simulink model "ASW_OBD"  (R2023a)
settings: configuration reference "cfg_FastTaskCodeGeneration_v01" (kept outside this file)
undefined symbols (not defined in the file): Cdbl_tiSlwTaskSmpTi
(part 1 of 2)
settings Model: DataDictionary=dd_foc_dictionary.sldd  EnableAccessToBaseWorkspace=off  Creator=WFYXQ  LastModifiedBy=xiaoqiang.yuan
settings ConfigSetRef: SourceName=cfg_FastTaskCodeGeneration_v01

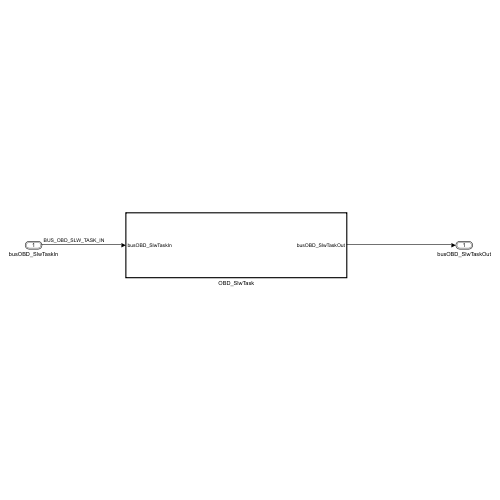
[thumbnail: Simulink's stored preview of the top-level diagram]
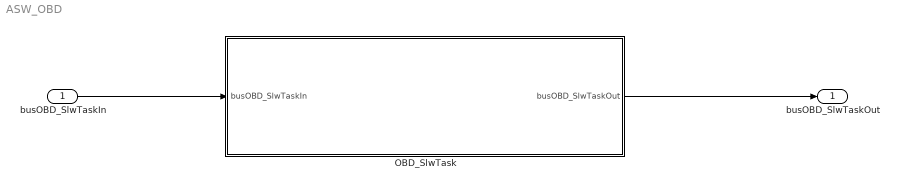
== system ASW_OBD ==
  busOBD_SlwTaskIn : Inport  OutDataTypeStr=Bus: BUS_OBD_SLW_TASK_IN  SampleTime=round(double(Cdbl_tiSlwTaskSmpTi),4)  BusOutputAsStruct=on
  OBD_SlwTask : Subsystem  TreatAsAtomicUnit=on  RTWFcnName=OBD_SlwTask
      settings: RTWSystemCode=Nonreusable function  RTWFcnNameOpts=User specified
  busOBD_SlwTaskOut : Outport  OutDataTypeStr=Bus: BUS_OBD_SLW_TASK_OUT  SampleTime=round(double(Cdbl_tiSlwTaskSmpTi),4)
  wires:
  busOBD_SlwTaskIn/1 -> OBD_SlwTask/1(busOBD_SlwTaskIn)
  OBD_SlwTask/1(busOBD_SlwTaskOut) -> busOBD_SlwTaskOut/1

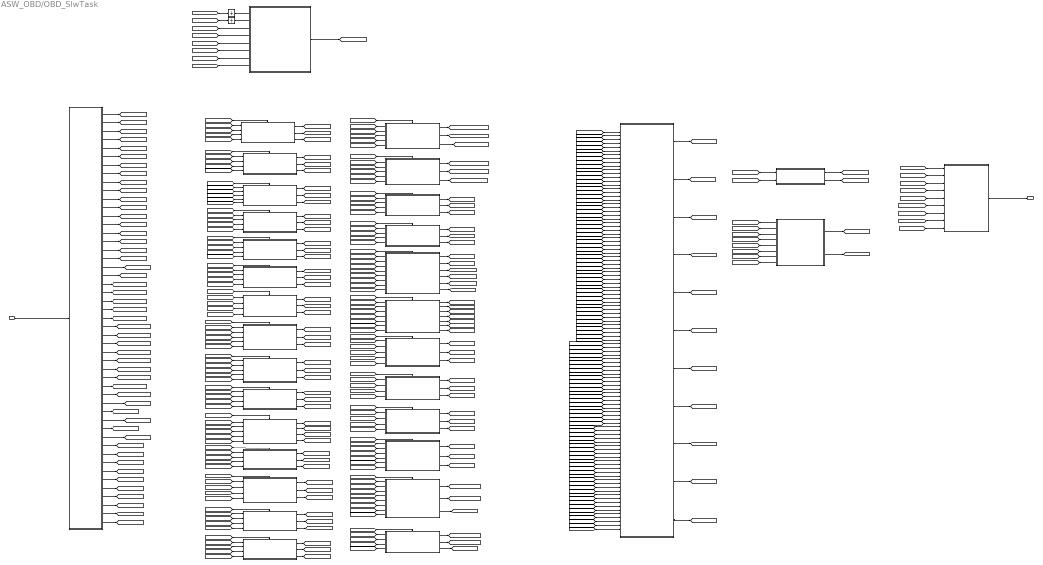
== system ASW_OBD/OBD_SlwTask ==
  note: FaultPreDiagnosis
  busOBD_SlwTaskIn : Inport
  Unit Delay : UnitDelay  SampleTime=-1  HasFrameUpgradeWarning=on
  Unit Delay1 : UnitDelay  SampleTime=-1  HasFrameUpgradeWarning=on
  rss_BattPwrHiLvl1Dia : Subsystem  ReferencedSubsystem=rss_BattPwrHiLvl1Dia
  rss_BusOffFaltDia : Subsystem  ReferencedSubsystem=rss_BusOffFaltDia
  rss_CRASHFaltDia : Subsystem  ReferencedSubsystem=rss_CrashFaltDia
  rss_ChipFaltDia : Subsystem  ReferencedSubsystem=rss_ChipFaltDia
  rss_ComFaltDia : Subsystem  ReferencedSubsystem=rss_ComFaltDia
  rss_CtlBrdVltgHiLvl1Dia : Subsystem  ReferencedSubsystem=rss_CtlBrdVltgHiLvl1Dia
  rss_CtlBrdVltgLoLvl1Dia : Subsystem  ReferencedSubsystem=rss_CtlBrdVltgLoLvl1Dia
  rss_FaltInfoMng : Subsystem  ReferencedSubsystem=rss_FaltInfoMng
  rss_FaltLevlCmpt : Subsystem  ReferencedSubsystem=rss_FaltLevlCmpt
  rss_FaltResp : Subsystem  ReferencedSubsystem=rss_FaltResp
  rss_GDVltgHiLvl1Dia : Subsystem  ReferencedSubsystem=rss_GDVltgHiLvl1Dia
  rss_GDVltgLoLvl1Dia : Subsystem  ReferencedSubsystem=rss_GDVltgLoLvl1Dia
  rss_HWOvrCurrDia : Subsystem  ReferencedSubsystem=rss_HWOvrCurrDia
  rss_MosOpnCirFaltDia : Subsystem  ReferencedSubsystem=rss_MosOpnCirFaltDia
  rss_MotoSpdHiLvl1Dia : Subsystem  ReferencedSubsystem=rss_MotoSpdHiLvl1Dia
  rss_MotoSpdLoLvl1Dia : Subsystem  ReferencedSubsystem=rss_MotoSpdLoLvl1Dia
  rss_MotoTempHiLvl1Dia : Subsystem  ReferencedSubsystem=rss_MotoTempHiLvl1Dia
  rss_MotoTempHiLvl2Dia : Subsystem  ReferencedSubsystem=rss_MotoTempHiLvl2Dia
  rss_MotoTempSensFaltDia : Subsystem  ReferencedSubsystem=rss_MotoTempSensFaltDia
  rss_NoLdDia : Subsystem  ReferencedSubsystem=rss_NoLdDia
  rss_PhCurrHiLvl1Dia : Subsystem  ReferencedSubsystem=rss_PhCurrHiLvl1Dia
  rss_PhCurrSensFaltDia : Subsystem  ReferencedSubsystem=rss_PhCurrSensFaltDia
  rss_PwrTubPCBTempHiLvl1Dia : Subsystem  ReferencedSubsystem=rss_PwrTubPCBTempHiLvl1Dia
  rss_PwrTubPCBTempHiLvl2Dia : Subsystem  ReferencedSubsystem=rss_PwrTubPCBTempHiLvl2Dia
  rss_PwrTubPCBTempSensFaltDia : Subsystem  ReferencedSubsystem=rss_PwrTubPCBTempSensFaltDia
  rss_SplyVltgHiLvl1Dia : Subsystem  ReferencedSubsystem=rss_SplyVltgHiLvl1Dia
  rss_SplyVltgLoLvl1Dia : Subsystem  ReferencedSubsystem=rss_SplyVltgLoLvl1Dia
  rss_SplyVltgLoLvl2Dia : Subsystem  ReferencedSubsystem=rss_SplyVltgLoLvl2Dia
  vrs_FaltEnFlgConf : Subsystem  Variant=on  VariantControlMode=label  VariantControl=Choice  LabelModeActiveChoice=cstSenlCtrlLbl
  vrs_MotoStallDia : Subsystem  Variant=on  VariantControlMode=label  VariantControl=Choice  LabelModeActiveChoice=cstHybrCtrlLbl
  vrs_PhiSensFaltDia : Subsystem  Variant=on  VariantControlMode=label  VariantControl=Choice  LabelModeActiveChoice=cstHybrCtrlLbl
  vrs_SlwTaskIn : Subsystem  Variant=on  VariantControlMode=label  VariantControl=cstSenlCtrlLbl  LabelModeActiveChoice=cstHybrCtrlLbl
  vrs_SlwTaskOut : Subsystem  Variant=on  VariantControlMode=label  VariantControl=Choice  LabelModeActiveChoice=cstHybrCtrlLbl
  busOBD_SlwTaskOut : Outport
  wires:
  vrs_SlwTaskOut/1(busOBD_SlwTaskOut) -> busOBD_SlwTaskOut/1  "busOBD_SlwTaskOut"
  [s16_nRmpRefElecSpd] -> rss_MotoSpdLoLvl1Dia/5
  [s16_nActElecSpd] -> rss_MotoSpdLoLvl1Dia/6
  [enm_stMotoSt] -> rss_MotoSpdLoLvl1Dia/4
  rss_PhCurrHiLvl1Dia/1 -> [bol_flgPhCurrHiLvl1Flg]
  rss_PhCurrHiLvl1Dia/2 -> [bol_flgPhCurrHiLvl1Occ]
  rss_ComFaltDia/1 -> [bol_flgComFaltFlg]
  rss_ComFaltDia/2 -> [bol_flgComFaltOcc]
  rss_BattPwrHiLvl1Dia/1 -> [bol_flgBattPwrHiLvl1Flg]
  rss_NoLdDia/1 -> [bol_flgNoLdFlg]
  rss_SplyVltgHiLvl1Dia/1 -> [bol_flgSplyVltgHiLvl1Flg]
  rss_MotoSpdHiLvl1Dia/1 -> [bol_flgMotoSpdHiLvl1Flg]
  rss_CtlBrdVltgLoLvl1Dia/1 -> [bol_flgCtlBrdVltgLoLvl1Flg]
  rss_FaltInfoMng/1 -> [busOBD_FaltSt]
  [busOBD_FaltSt] -> vrs_SlwTaskOut/1(busOBD_FaltSt)
  [bol_FaltSt] -> rss_FaltLevlCmpt/1
  rss_FaltInfoMng/2 -> [bol_FaltSt]
  [busOBD_FaltSt] -> Unit Delay/1
  [bol_enFaltEnFlg] -> rss_PhCurrHiLvl1Dia/1
  rss_FaltInfoMng/4 -> [u8_stFaltCyclDiaCt]
  rss_FaltInfoMng/5 -> [bol_enFaltRcvEnFlg]
  rss_FaltInfoMng/6 -> [bol_enFaltMngEnFlg]
  [u8_stFaltCyclDiaCt] -> rss_PhCurrHiLvl1Dia/2
  [bol_enFaltRcvEnFlg] -> rss_PhCurrHiLvl1Dia/3
  rss_FaltLevlCmpt/1 -> [u8_stFaltLvl]
  rss_FaltLevlCmpt/2 -> [u8_stMaxFaltLvl]
  rss_FaltInfoMng/7 -> [u8_stFaltLvlCt]
  [u8_stFaltLvlCt] -> rss_FaltLevlCmpt/2
  [u8_stFaltLvl] -> rss_FaltResp/1
  [u8_stMaxFaltLvl] -> rss_FaltResp/2
  rss_FaltResp/1 -> [s16_nFaltRefMechSpd]
  rss_FaltResp/2 -> [s16_trqFaltRefTqLim]
  [u8_ctMotoStallCyclAcc] -> rss_FaltResp/3
  [bol_enFaltEnFlg] -> rss_SplyVltgHiLvl1Dia/1
  [u8_stFaltCyclDiaCt] -> rss_SplyVltgHiLvl1Dia/2
  [bol_enFaltRcvEnFlg] -> rss_SplyVltgHiLvl1Dia/3
  [bol_enFaltEnFlg] -> rss_ComFaltDia/1
  [u8_stFaltCyclDiaCt] -> rss_ComFaltDia/2
  [bol_enFaltRcvEnFlg] -> rss_ComFaltDia/3
  [bol_enFaltEnFlg] -> rss_NoLdDia/1
  [u8_stFaltCyclDiaCt] -> rss_NoLdDia/2
  [bol_enFaltRcvEnFlg] -> rss_NoLdDia/3
  [s16_nActElecSpd] -> rss_NoLdDia/5
  [s16_ampActPhCurrAmp] -> rss_PhCurrHiLvl1Dia/4
  [u16_uSplyVltg] -> rss_SplyVltgHiLvl1Dia/4
  [u8_ctLossNoData] -> rss_ComFaltDia/4
  [u8_ctComRolCnt] -> rss_ComFaltDia/5
  [s16_ampActPhCurrAmp] -> rss_NoLdDia/4
  [bol_enFaltEnFlg] -> rss_MotoSpdLoLvl1Dia/1
  [u8_stFaltCyclDiaCt] -> rss_MotoSpdLoLvl1Dia/2
  [bol_enFaltRcvEnFlg] -> rss_MotoSpdLoLvl1Dia/3
  [u8_ctMotoStallCyclDiaCnt] -> rss_FaltResp/4
  [u8_stMaxFaltLvl] -> vrs_SlwTaskOut/2(u8_stMaxFaltLvl)
  [s16_nFaltRefMechSpd] -> vrs_SlwTaskOut/3(s16_nFaltRefMechSpd)
  [s16_trqFaltRefTqLim] -> vrs_SlwTaskOut/4(s16_trqFaltRefTqLim)
  rss_MotoSpdLoLvl1Dia/1 -> [bol_flgMotoSpdLoLvl1Flg]
  [bol_enFaltEnFlg] -> rss_CtlBrdVltgLoLvl1Dia/1
  [u16_uCtlBrdVltg] -> rss_CtlBrdVltgLoLvl1Dia/4
  [u8_stFaltCyclDiaCt] -> rss_CtlBrdVltgLoLvl1Dia/2
  [bol_enFaltRcvEnFlg] -> rss_CtlBrdVltgLoLvl1Dia/3
  rss_FaltInfoMng/8 -> [bol_flgFstSdlEn]
  rss_FaltInfoMng/9 -> [bol_flgSlwSdlEn]
  [bol_flgFstSdlEn] -> rss_CtlBrdVltgLoLvl1Dia/Enable
  rss_CtlBrdVltgLoLvl1Dia/2 -> [bol_flgCtlBrdVltgLoLvl1Occ]
  [u8_stFaltCyclDiaCt] -> rss_CtlBrdVltgHiLvl1Dia/2
  [bol_flgFstSdlEn] -> rss_CtlBrdVltgHiLvl1Dia/Enable
  [bol_enFaltEnFlg] -> rss_CtlBrdVltgHiLvl1Dia/1
  [bol_enFaltRcvEnFlg] -> rss_CtlBrdVltgHiLvl1Dia/3
  rss_CtlBrdVltgHiLvl1Dia/2 -> [bol_flgCtlBrdVltgHiLvl1Occ]
  rss_CtlBrdVltgHiLvl1Dia/1 -> [bol_flgCtlBrdVltgHiLvl1Flg]
  [u16_uCtlBrdVltg] -> rss_CtlBrdVltgHiLvl1Dia/4
  [bol_flgFstSdlEn] -> rss_PhCurrHiLvl1Dia/Enable
  [bol_flgFstSdlEn] -> rss_HWOvrCurrDia/Enable
  [bol_enFaltEnFlg] -> rss_HWOvrCurrDia/1
  [u8_stFaltCyclDiaCt] -> rss_HWOvrCurrDia/2
  [bol_enFaltRcvEnFlg] -> rss_HWOvrCurrDia/3
  [bol_flgHWOvrCurrFalt] -> rss_HWOvrCurrDia/4
  rss_HWOvrCurrDia/1 -> [bol_flgHWOvrCurrFlg]
  rss_HWOvrCurrDia/2 -> [bol_flgHWOvrCurrOcc]
  [bol_flgFstSdlEn] -> rss_SplyVltgLoLvl1Dia/Enable
  [bol_enFaltEnFlg] -> rss_SplyVltgLoLvl1Dia/1
  [u8_stFaltCyclDiaCt] -> rss_SplyVltgLoLvl1Dia/2
  [bol_enFaltRcvEnFlg] -> rss_SplyVltgLoLvl1Dia/3
  [u16_uSplyVltg] -> rss_SplyVltgLoLvl1Dia/4
  rss_SplyVltgLoLvl1Dia/1 -> [bol_flgSplyVltgLoLvl1Flg]
  rss_SplyVltgLoLvl1Dia/2 -> [bol_flgSplyVltgLoLvl1Occ]
  [bol_flgFstSdlEn] -> rss_SplyVltgLoLvl2Dia/Enable
  [bol_enFaltEnFlg] -> rss_SplyVltgLoLvl2Dia/1
  [u8_stFaltCyclDiaCt] -> rss_SplyVltgLoLvl2Dia/2
  [bol_enFaltRcvEnFlg] -> rss_SplyVltgLoLvl2Dia/3
  [u16_uSplyVltg] -> rss_SplyVltgLoLvl2Dia/4
  rss_SplyVltgLoLvl2Dia/1 -> [bol_flgSplyVltgLoLvl2Flg]
  rss_SplyVltgLoLvl2Dia/2 -> [bol_flgSplyVltgLoLvl2Occ]
  [bol_flgFstSdlEn] -> rss_SplyVltgHiLvl1Dia/Enable
  rss_SplyVltgHiLvl1Dia/2 -> [bol_flgSplyVltgHiLvl1Occ]
  [bol_enFaltEnFlg] -> rss_PwrTubPCBTempHiLvl1Dia/1
  [u8_stFaltCyclDiaCt] -> rss_PwrTubPCBTempHiLvl1Dia/2
  [bol_enFaltRcvEnFlg] -> rss_PwrTubPCBTempHiLvl1Dia/3
  [u8_tPwrTubTemp] -> rss_PwrTubPCBTempHiLvl1Dia/4
  [u8_tPCBTempSubs] -> rss_PwrTubPCBTempHiLvl1Dia/5
  [bol_flgSlwSdlEn] -> rss_PwrTubPCBTempHiLvl1Dia/Enable
  rss_PwrTubPCBTempHiLvl1Dia/1 -> [bol_flgPwrTubPCBTempHiLvl1Flg]
  rss_PwrTubPCBTempHiLvl1Dia/2 -> [bol_flgPwrTubPCBTempHiLvl1Occ]
  [bol_flgSlwSdlEn] -> rss_PwrTubPCBTempHiLvl2Dia/Enable
  [bol_enFaltEnFlg] -> rss_PwrTubPCBTempHiLvl2Dia/1
  [u8_stFaltCyclDiaCt] -> rss_PwrTubPCBTempHiLvl2Dia/2
  [bol_enFaltRcvEnFlg] -> rss_PwrTubPCBTempHiLvl2Dia/3
  [u8_tPwrTubTemp] -> rss_PwrTubPCBTempHiLvl2Dia/4
  [u8_tPCBTempSubs] -> rss_PwrTubPCBTempHiLvl2Dia/5
  rss_PwrTubPCBTempHiLvl2Dia/1 -> [bol_flgPwrTubPCBTempHiLvl2Flg]
  rss_PwrTubPCBTempHiLvl2Dia/2 -> [bol_flgPwrTubPCBTempHiLvl2Occ]
  [bol_enFaltEnFlg] -> rss_MotoTempHiLvl1Dia/1
  [u8_stFaltCyclDiaCt] -> rss_MotoTempHiLvl1Dia/2
  [bol_enFaltRcvEnFlg] -> rss_MotoTempHiLvl1Dia/3
  [u8_tMotoTemp] -> rss_MotoTempHiLvl1Dia/4
  [bol_flgSlwSdlEn] -> rss_MotoTempHiLvl1Dia/Enable
  rss_MotoTempHiLvl1Dia/1 -> [bol_flgMotoTempHiLvl1Flg]
  rss_MotoTempHiLvl1Dia/2 -> [bol_flgMotoTempHiLvl1Occ]
  [u8_tMotoTemp] -> rss_MotoTempHiLvl2Dia/4
  [bol_flgSlwSdlEn] -> rss_MotoTempHiLvl2Dia/Enable
  [u8_stFaltCyclDiaCt] -> rss_MotoTempHiLvl2Dia/2
  rss_MotoTempHiLvl2Dia/1 -> [bol_flgMotoTempHiLvl2Flg]
  [bol_enFaltEnFlg] -> rss_MotoTempHiLvl2Dia/1
  [bol_enFaltRcvEnFlg] -> rss_MotoTempHiLvl2Dia/3
  rss_MotoTempHiLvl2Dia/2 -> [bol_flgMotoTempHiLvl2Occ]
  [bol_flgFstSdlEn] -> rss_NoLdDia/Enable
  rss_NoLdDia/2 -> [bol_flgNoLdOcc]
  [s16_pwrSplyElecPwr] -> rss_BattPwrHiLvl1Dia/4
  [bol_enFaltEnFlg] -> rss_BattPwrHiLvl1Dia/1
  [u8_stFaltCyclDiaCt] -> rss_BattPwrHiLvl1Dia/2
  [bol_enFaltRcvEnFlg] -> rss_BattPwrHiLvl1Dia/3
  [bol_flgSlwSdlEn] -> rss_BattPwrHiLvl1Dia/Enable
  rss_BattPwrHiLvl1Dia/2 -> [bol_flgBattPwrHiLvl1Occ]
  rss_MotoSpdLoLvl1Dia/2 -> [bol_flgMotoSpdLoLvl1Occ]
  [bol_flgSlwSdlEn] -> rss_MotoSpdLoLvl1Dia/Enable
  rss_MotoSpdHiLvl1Dia/2 -> [bol_flgMotoSpdHiLvl1Occ]
  [bol_enFaltRcvEnFlg] -> rss_MotoSpdHiLvl1Dia/3
  [u8_stFaltCyclDiaCt] -> rss_MotoSpdHiLvl1Dia/2
  [bol_enFaltEnFlg] -> rss_MotoSpdHiLvl1Dia/1
  [bol_flgSlwSdlEn] -> rss_MotoSpdHiLvl1Dia/Enable
  [s16_nActElecSpd] -> rss_MotoSpdHiLvl1Dia/4
  [bol_flgGDVltgHiLvl1] -> rss_GDVltgHiLvl1Dia/4
  rss_GDVltgHiLvl1Dia/1 -> [bol_flgGDVltgHiLvl1Flg]
  rss_GDVltgHiLvl1Dia/2 -> [bol_flgGDVltgHiLvl1Occ]
  [bol_enFaltRcvEnFlg] -> rss_GDVltgHiLvl1Dia/3
  [bol_enFaltEnFlg] -> rss_GDVltgHiLvl1Dia/1
  [bol_flgFstSdlEn] -> rss_GDVltgHiLvl1Dia/Enable
  [u8_stFaltCyclDiaCt] -> rss_GDVltgHiLvl1Dia/2
  rss_GDVltgLoLvl1Dia/2 -> [bol_flgGDVltgLoLvl1Occ]
  [bol_flgFstSdlEn] -> rss_GDVltgLoLvl1Dia/Enable
  [bol_enFaltRcvEnFlg] -> rss_GDVltgLoLvl1Dia/3
  [u8_stFaltCyclDiaCt] -> rss_GDVltgLoLvl1Dia/2
  [bol_flgGDVltgLoLvl1] -> rss_GDVltgLoLvl1Dia/4
  [bol_enFaltEnFlg] -> rss_GDVltgLoLvl1Dia/1
  rss_GDVltgLoLvl1Dia/1 -> [bol_flgGDVltgLoLvl1Flg]
  rss_ChipFaltDia/1 -> [bol_flgChipFaltFlg]
  [bol_enFaltEnFlg] -> rss_ChipFaltDia/1
  [u8_stFaltCyclDiaCt] -> rss_ChipFaltDia/2
  [bol_enFaltRcvEnFlg] -> rss_ChipFaltDia/3
  [bol_flgChipFalt] -> rss_ChipFaltDia/4
  [bol_flgFstSdlEn] -> rss_ChipFaltDia/Enable
  rss_ChipFaltDia/2 -> [bol_flgChipFaltOcc]
  [u16_uADActPhCurr] -> rss_PhCurrSensFaltDia/4
  [bol_flgFstSdlEn] -> rss_PhCurrSensFaltDia/Enable
  [bol_enFaltEnFlg] -> rss_PhCurrSensFaltDia/1
  [u8_stFaltCyclDiaCt] -> rss_PhCurrSensFaltDia/2
  [bol_enFaltRcvEnFlg] -> rss_PhCurrSensFaltDia/3
  rss_PhCurrSensFaltDia/1 -> [bol_flgPhCurrSensFaltFlg]
  rss_PhCurrSensFaltDia/2 -> [bol_flgPhCurrSensFaltOcc]
  rss_PwrTubPCBTempSensFaltDia/1 -> [bol_flgPwrTubPCBTempSensFaltFlg]
  rss_PwrTubPCBTempSensFaltDia/2 -> [bol_flgPwrTubPCBTempSensFaltOcc]
  [bol_flgSlwSdlEn] -> rss_PwrTubPCBTempSensFaltDia/Enable
  [bol_enFaltEnFlg] -> rss_PwrTubPCBTempSensFaltDia/1
  [u8_stFaltCyclDiaCt] -> rss_PwrTubPCBTempSensFaltDia/2
  [bol_enFaltRcvEnFlg] -> rss_PwrTubPCBTempSensFaltDia/3
  [u16_uADPwrTubTemp] -> rss_PwrTubPCBTempSensFaltDia/4
  [u16_uADPCBTemp] -> rss_PwrTubPCBTempSensFaltDia/5
  [u16_uADMotoTemp] -> rss_MotoTempSensFaltDia/4
  [bol_enFaltRcvEnFlg] -> rss_MotoTempSensFaltDia/3
  [u8_stFaltCyclDiaCt] -> rss_MotoTempSensFaltDia/2
  [bol_enFaltEnFlg] -> rss_MotoTempSensFaltDia/1
  [bol_flgSlwSdlEn] -> rss_MotoTempSensFaltDia/Enable
  rss_MotoTempSensFaltDia/1 -> [bol_flgMotoTempSensFaltFlg]
  rss_MotoTempSensFaltDia/2 -> [bol_flgMotoTempSensFaltOcc]
  [bol_flgComSdlEn] -> rss_ComFaltDia/Enable
  [bol_flgPhCurrHiLvl1Flg] -> rss_FaltInfoMng/1
  [bol_flgHWOvrCurrFlg] -> rss_FaltInfoMng/2
  [bol_flgSplyVltgLoLvl1Flg] -> rss_FaltInfoMng/3
  [bol_flgSplyVltgLoLvl2Flg] -> rss_FaltInfoMng/4
  [bol_flgSplyVltgHiLvl1Flg] -> rss_FaltInfoMng/5
  [bol_flgPwrTubPCBTempHiLvl1Flg] -> rss_FaltInfoMng/6
  [bol_flgPwrTubPCBTempHiLvl2Flg] -> rss_FaltInfoMng/7
  [bol_flgMotoTempHiLvl1Flg] -> rss_FaltInfoMng/8
  [bol_flgMotoTempHiLvl2Flg] -> rss_FaltInfoMng/9
  [bol_flgComFaltFlg] -> rss_FaltInfoMng/10
  [bol_flgMotoStallPermFlg] -> rss_FaltInfoMng/11
  [bol_flgMotoStallTmpFlg] -> rss_FaltInfoMng/12
  [bol_flgNoLdFlg] -> rss_FaltInfoMng/13
  [bol_flgBattPwrHiLvl1Flg] -> rss_FaltInfoMng/14
  [bol_flgMotoSpdHiLvl1Flg] -> rss_FaltInfoMng/15
  [bol_flgMotoSpdLoLvl1Flg] -> rss_FaltInfoMng/16
  [bol_flgCtlBrdVltgLoLvl1Flg] -> rss_FaltInfoMng/17
  [bol_flgCtlBrdVltgHiLvl1Flg] -> rss_FaltInfoMng/18
  [bol_flgGDVltgLoLvl1Flg] -> rss_FaltInfoMng/19
  [bol_flgGDVltgHiLvl1Flg] -> rss_FaltInfoMng/20
  [bol_flgChipFaltFlg] -> rss_FaltInfoMng/21
  [bol_flgPhiSensFaltFlg] -> rss_FaltInfoMng/22
  [bol_flgPhCurrSensFaltFlg] -> rss_FaltInfoMng/23
  [bol_flgPwrTubPCBTempSensFaltFlg] -> rss_FaltInfoMng/24
  [bol_flgMotoTempSensFaltFlg] -> rss_FaltInfoMng/25
  [bol_flgPhCurrHiLvl1Occ] -> rss_FaltInfoMng/29
  [bol_flgHWOvrCurrOcc] -> rss_FaltInfoMng/30
  [bol_flgSplyVltgLoLvl1Occ] -> rss_FaltInfoMng/31
  [bol_flgSplyVltgLoLvl2Occ] -> rss_FaltInfoMng/32
  [bol_flgSplyVltgHiLvl1Occ] -> rss_FaltInfoMng/33
  [bol_flgPwrTubPCBTempHiLvl1Occ] -> rss_FaltInfoMng/34
  [bol_flgPwrTubPCBTempHiLvl2Occ] -> rss_FaltInfoMng/35
  [bol_flgMotoTempHiLvl1Occ] -> rss_FaltInfoMng/36
  [bol_flgMotoTempHiLvl2Occ] -> rss_FaltInfoMng/37
  [bol_flgComFaltOcc] -> rss_FaltInfoMng/38
  [bol_flgMotoStallOcc] -> rss_FaltInfoMng/39
  [bol_flgMotoStallOcc] -> rss_FaltInfoMng/40
  [bol_flgNoLdOcc] -> rss_FaltInfoMng/41
  [bol_flgBattPwrHiLvl1Occ] -> rss_FaltInfoMng/42
  [bol_flgMotoSpdHiLvl1Occ] -> rss_FaltInfoMng/43
  [bol_flgMotoSpdLoLvl1Occ] -> rss_FaltInfoMng/44
  [bol_flgCtlBrdVltgLoLvl1Occ] -> rss_FaltInfoMng/45
  [bol_flgCtlBrdVltgHiLvl1Occ] -> rss_FaltInfoMng/46
  [bol_flgGDVltgLoLvl1Occ] -> rss_FaltInfoMng/47
  [bol_flgGDVltgHiLvl1Occ] -> rss_FaltInfoMng/48
  [bol_flgChipFaltOcc] -> rss_FaltInfoMng/49
  [bol_flgPhiSensFaltOcc] -> rss_FaltInfoMng/50
  [bol_flgPhCurrSensFaltOcc] -> rss_FaltInfoMng/51
  [bol_flgPwrTubPCBTempSensFaltOcc] -> rss_FaltInfoMng/52
  [bol_flgMotoTempSensFaltOcc] -> rss_FaltInfoMng/53
  rss_FaltInfoMng/3 -> [bus_FaltStOcc]
  [bus_FaltStOcc] -> Unit Delay1/1
  [busOBD_FaltSt] -> rss_FaltResp/5
  [bol_flgSlwSdlEn] -> rss_FaltResp/6
  [u16_uSplyVltg] -> rss_FaltInfoMng/57
  [s16_nRmpRefElecSpd] -> rss_FaltInfoMng/58
  [u8_tPCBTemp] -> rss_FaltInfoMng/59
  [u8_tMotoTemp] -> rss_FaltInfoMng/60
  [u8_tPwrTubTemp] -> rss_FaltInfoMng/61
  [u16_uCtlBrdVltg] -> rss_FaltInfoMng/62
  [s16_iActPhCurr] -> rss_FaltInfoMng/63
  [enm_stMotoSt] -> rss_FaltInfoMng/64
  [s16_iEstSplyCurr] -> rss_FaltInfoMng/65
  [s16_iRefDaxQaxCurr] -> rss_FaltInfoMng/66
  [s16_iActDaxQaxCurr] -> rss_FaltInfoMng/67
  [s16_nActElecSpd] -> rss_FaltInfoMng/68
  [bol_flgShOffFlg] -> rss_FaltInfoMng/69
  [bol_enFaltInfoClrUDS14] -> rss_FaltInfoMng/70
  [u16_vVehSpd] -> rss_FaltInfoMng/71
  [u32_disOde] -> rss_FaltInfoMng/72
  [u32_tiStamHi] -> rss_FaltInfoMng/73
  [u32_tiStamLo] -> rss_FaltInfoMng/74
  [u8_psiOilFlow] -> rss_FaltInfoMng/75
  [u8_tOilTemp] -> rss_FaltInfoMng/76
  [bol_enPosSCDCalibEnFlg] -> rss_FaltInfoMng/77
  [u8_psiUpLimOilFlow] -> rss_FaltInfoMng/78
  [bol_flgFstSdlEn] -> rss_BusOffFaltDia/Enable
  [bol_flgBusOffFaltRaw] -> rss_BusOffFaltDia/4
  [bol_enFaltRcvEnFlg] -> rss_BusOffFaltDia/3
  [u8_stFaltCyclDiaCt] -> rss_BusOffFaltDia/2
  [bol_enFaltEnFlg] -> rss_BusOffFaltDia/1
  rss_BusOffFaltDia/2 -> [bol_flgBusOffFaltOcc]
  rss_BusOffFaltDia/1 -> [bol_flgBusOffFaltFlg]
  [bol_flgBusOffFaltOcc] -> rss_FaltInfoMng/54
  [bol_flgBusOffFaltFlg] -> rss_FaltInfoMng/26
  [bol_flgCRCFaltRaw] -> rss_ComFaltDia/6
  [bol_flgMesgLngthFaltRaw] -> rss_ComFaltDia/7
  [s16_nComRefMechSpd] -> rss_ComFaltDia/8
  rss_FaltInfoMng/10 -> [bol_flgComSdlEn]
  [bol_enFaltEnFlg] -> vrs_MotoStallDia/1(bol_enFaltEnFlg)
  [u8_stFaltCyclDiaCt] -> vrs_MotoStallDia/2(u8_stFaltCyclDiaCt)
  [bol_enFaltRcvEnFlg] -> vrs_MotoStallDia/3(bol_enFaltRcvEnFlg)
  [s16_nRmpRefElecSpd] -> vrs_MotoStallDia/4(s16_nRmpRefElecSpd)
  [s16_nActElecSpd] -> vrs_MotoStallDia/5(s16_nActElecSpd)
  [bol_flgFstSdlEn] -> vrs_MotoStallDia/Enable
  vrs_MotoStallDia/1(bol_flgMotoStallTmpFlg) -> [bol_flgMotoStallTmpFlg]
  vrs_MotoStallDia/2(bol_flgMotoStallPermFlg) -> [bol_flgMotoStallPermFlg]
  vrs_MotoStallDia/3(u8_ctMotoStallCyclAcc) -> [u8_ctMotoStallCyclAcc]
  vrs_MotoStallDia/4(bol_flgMotoStallOcc) -> [bol_flgMotoStallOcc]
  vrs_MotoStallDia/5(u8_ctMotoStallCyclDiaCnt) -> [u8_ctMotoStallCyclDiaCnt]
  [u16_psiEstPermMagFlx] -> vrs_MotoStallDia/6(u16_psiEstPermMagFlx)
  Unit Delay/1 -> vrs_FaltEnFlgConf/1(busOBD_FaltSt)
  Unit Delay1/1 -> vrs_FaltEnFlgConf/2(bus_FaltStOcc)
  [bol_enFaltMngEnFlg] -> vrs_FaltEnFlgConf/3(bol_enFaltMngEnFlg)
  [enm_stSysSt] -> vrs_FaltEnFlgConf/4(enm_stSysSt)
  [s16_nComRefMechSpd] -> vrs_FaltEnFlgConf/5(s16_nComRefMechSpd)
  [bol_flgFaltEnFlgUDS85] -> vrs_FaltEnFlgConf/6(bol_flgFaltEnFlgUDS85)
  [bol_flgWBSSt] -> vrs_FaltEnFlgConf/7(bol_flgWBSSt)
  [u16_uCtlBrdVltg] -> vrs_FaltEnFlgConf/8(u16_uCtlBrdVltg)
  vrs_FaltEnFlgConf/1(bol_enFaltEnFlg) -> [bol_enFaltEnFlg]
  busOBD_SlwTaskIn/1 -> vrs_SlwTaskIn/1(busOBD_SlwTaskIn)  "busOBD_SlwTaskIn"
  vrs_SlwTaskIn/1(s16_nRmpRefElecSpd) -> [s16_nRmpRefElecSpd]
  vrs_SlwTaskIn/2(s16_nActElecSpd) -> [s16_nActElecSpd]
  vrs_SlwTaskIn/3(enm_stMotoSt) -> [enm_stMotoSt]
  vrs_SlwTaskIn/4(s16_ampActPhCurrAmp) -> [s16_ampActPhCurrAmp]
  vrs_SlwTaskIn/5(u16_uSplyVltg) -> [u16_uSplyVltg]
  vrs_SlwTaskIn/6(u8_tPwrTubTemp) -> [u8_tPwrTubTemp]
  vrs_SlwTaskIn/7(u8_tPCBTemp) -> [u8_tPCBTemp]
  vrs_SlwTaskIn/8(u8_tMotoTemp) -> [u8_tMotoTemp]
  vrs_SlwTaskIn/9(u8_ctLossNoData) -> [u8_ctLossNoData]
  vrs_SlwTaskIn/10(u8_ctComRolCnt) -> [u8_ctComRolCnt]
  vrs_SlwTaskIn/11(u16_uCtlBrdVltg) -> [u16_uCtlBrdVltg]
  vrs_SlwTaskIn/12(enm_stSysSt) -> [enm_stSysSt]
  vrs_SlwTaskIn/13(bol_flgHWOvrCurrFalt) -> [bol_flgHWOvrCurrFalt]
  vrs_SlwTaskIn/14(bol_flgChipFalt) -> [bol_flgChipFalt]
  vrs_SlwTaskIn/15(bol_flgPhiSensFalt) -> [bol_flgPhiSensFalt]
  vrs_SlwTaskIn/16(u16_uADActPhCurr) -> [u16_uADActPhCurr]
  vrs_SlwTaskIn/17(u16_uADPwrTubTemp) -> [u16_uADPwrTubTemp]
  vrs_SlwTaskIn/18(u16_uADPCBTemp) -> [u16_uADPCBTemp]
  vrs_SlwTaskIn/19(u16_uADMotoTemp) -> [u16_uADMotoTemp]
  vrs_SlwTaskIn/20(s16_pwrSplyElecPwr) -> [s16_pwrSplyElecPwr]
  vrs_SlwTaskIn/21(s16_iActPhCurr) -> [s16_iActPhCurr]
  vrs_SlwTaskIn/22(s16_iEstSplyCurr) -> [s16_iEstSplyCurr]
  vrs_SlwTaskIn/23(s16_iRefDaxQaxCurr) -> [s16_iRefDaxQaxCurr]
  vrs_SlwTaskIn/24(s16_iActDaxQaxCurr) -> [s16_iActDaxQaxCurr]
  vrs_SlwTaskIn/25(bol_flgShOffFlg) -> [bol_flgShOffFlg]
  vrs_SlwTaskIn/26(bol_enFaltInfoClrUDS14) -> [bol_enFaltInfoClrUDS14]
  vrs_SlwTaskIn/27(u16_vVehSpd) -> [u16_vVehSpd]
  vrs_SlwTaskIn/28(u32_disOde) -> [u32_disOde]
  vrs_SlwTaskIn/29(u32_tiStamHi) -> [u32_tiStamHi]
  vrs_SlwTaskIn/30(u32_tiStamLo) -> [u32_tiStamLo]
  vrs_SlwTaskIn/31(u8_psiOilFlow) -> [u8_psiOilFlow]
  vrs_SlwTaskIn/32(u8_tOilTemp) -> [u8_tOilTemp]
  vrs_SlwTaskIn/33(bol_enPosSCDCalibEnFlg) -> [bol_enPosSCDCalibEnFlg]
  vrs_SlwTaskIn/34(u8_psiUpLimOilFlow) -> [u8_psiUpLimOilFlow]
  vrs_SlwTaskIn/35(bol_flgBusOffFaltRaw) -> [bol_flgBusOffFaltRaw]
  vrs_SlwTaskIn/36(bol_flgFaltEnFlgUDS85) -> [bol_flgFaltEnFlgUDS85]
  vrs_SlwTaskIn/37(bol_flgWBSSt) -> [bol_flgWBSSt]
  vrs_SlwTaskIn/38(bol_flgCRCFaltRaw) -> [bol_flgCRCFaltRaw]
  vrs_SlwTaskIn/39(bol_flgMesgLngthFaltRaw) -> [bol_flgMesgLngthFaltRaw]
  vrs_SlwTaskIn/40(s16_nComRefMechSpd) -> [s16_nComRefMechSpd]
  vrs_SlwTaskIn/41(u16_psiEstPermMagFlx) -> [u16_psiEstPermMagFlx]
  [bol_enFaltEnFlg] -> vrs_PhiSensFaltDia/1(bol_enFaltEnFlg)
  [u8_stFaltCyclDiaCt] -> vrs_PhiSensFaltDia/2(u8_stFaltCyclDiaCt)
  [bol_enFaltRcvEnFlg] -> vrs_PhiSensFaltDia/3(bol_enFaltRcvEnFlg)
  [bol_flgPhiSensFalt] -> vrs_PhiSensFaltDia/4(bol_flgPhiSensFalt)
  [bol_flgFstSdlEn] -> vrs_PhiSensFaltDia/Enable
  vrs_PhiSensFaltDia/1(bol_flgPhiSensFaltFlg) -> [bol_flgPhiSensFaltFlg]
  vrs_PhiSensFaltDia/2(bol_flgPhiSensFaltOcc) -> [bol_flgPhiSensFaltOcc]
  vrs_PhiSensFaltDia/3(bol_flgPhiSensFaltRawFlg) -> [bol_flgPhiSensFaltRawFlg]
  [enm_modeAgEvalMode] -> vrs_PhiSensFaltDia/5(enm_modeAgEvalMode)
  [enm_modeAgEvalMode] -> vrs_MotoStallDia/7(enm_modeAgEvalMode)
  [bol_flgPhiSensFaltRawFlg] -> vrs_SlwTaskOut/5(bol_flgPhiSensFaltRawFlg)
  vrs_SlwTaskIn/42(enm_modeAgEvalMode) -> [enm_modeAgEvalMode]
  [enm_stSysSt] -> rss_FaltResp/7
  [bol_enFaltRcvEnFlg] -> rss_CRASHFaltDia/3
  [bol_flgCrashFalt] -> rss_CRASHFaltDia/4
  [u8_stFaltCyclDiaCt] -> rss_CRASHFaltDia/2
  [bol_enFaltEnFlg] -> rss_CRASHFaltDia/1
  [bol_flgFstSdlEn] -> rss_CRASHFaltDia/Enable
  rss_CRASHFaltDia/1 -> [bol_flgCrashFaltFlg]
  rss_CRASHFaltDia/2 -> [bol_flgCrashFaltOcc]
  [bol_flgCrashFaltFlg] -> rss_FaltInfoMng/27
  [bol_flgCrashFaltOcc] -> rss_FaltInfoMng/55
  [u16_uSplyVltg] -> rss_FaltResp/8
  vrs_SlwTaskIn/43(bol_flgCrashFalt) -> [bol_flgCrashFalt]
  vrs_SlwTaskIn/45(bol_flgGDVltgLoLvl1) -> [bol_flgGDVltgLoLvl1]
  vrs_SlwTaskIn/44(bol_flgGDVltgHiLvl1) -> [bol_flgGDVltgHiLvl1]
  [u8_tPwrTubTemp] -> rss_PwrTubPCBTempSensFaltDia/6
  [u8_tPCBTemp] -> rss_PwrTubPCBTempSensFaltDia/7
  [u8_tMCUTemp] -> rss_PwrTubPCBTempSensFaltDia/8
  vrs_SlwTaskIn/46(u8_tMCUTemp) -> [u8_tMCUTemp]
  vrs_SlwTaskIn/47(u8_tPCBTempSubs) -> [u8_tPCBTempSubs]
  [u16_uGDVltg] -> rss_GDVltgHiLvl1Dia/5
  [u16_uGDVltg] -> rss_GDVltgLoLvl1Dia/5
  vrs_SlwTaskIn/48(u16_uGDVltg) -> [u16_uGDVltg]
  rss_ComFaltDia/3 -> [bol_flgComNodeLosFaltDeb]
  rss_ComFaltDia/4 -> [bol_flgComRolCntFaltDeb]
  rss_ComFaltDia/5 -> [bol_flgCRCFaltDeb]
  [bol_flgComNodeLosFaltDeb] -> vrs_SlwTaskOut/6(bol_flgComNodeLosFaltDeb)
  [bol_flgComRolCntFaltDeb] -> vrs_SlwTaskOut/7(bol_flgComRolCntFaltDeb)
  [bol_flgCRCFaltDeb] -> vrs_SlwTaskOut/8(bol_flgCRCFaltDeb)
  [bol_flgMosOpnCirFalt] -> rss_MosOpnCirFaltDia/4
  [bol_enFaltEnFlg] -> rss_MosOpnCirFaltDia/1
  [bol_enFaltRcvEnFlg] -> rss_MosOpnCirFaltDia/3
  rss_MosOpnCirFaltDia/1 -> [bol_flgMosOpnCirFaltFlg]
  rss_MosOpnCirFaltDia/2 -> [bol_flgMosOpnCirFaltOcc]
  [u8_stFaltCyclDiaCt] -> rss_MosOpnCirFaltDia/2
  [bol_flgFstSdlEn] -> rss_MosOpnCirFaltDia/Enable
  [bol_flgMosOpnCirFaltFlg] -> rss_FaltInfoMng/28
  [bol_flgMosOpnCirFaltOcc] -> rss_FaltInfoMng/56
  [bol_flgPhCurrHiLvl1Tmp] -> rss_FaltInfoMng/79
  [bol_flgHWOvrCurrTmp] -> rss_FaltInfoMng/80
  [bol_flgSplyVltgLoLvl1Tmp] -> rss_FaltInfoMng/81
  [bol_flgSplyVltgLoLvl2Tmp] -> rss_FaltInfoMng/82
  [bol_flgSplyVltgHiLvl1Tmp] -> rss_FaltInfoMng/83
  [bol_flgPwrTubPCBTempHiLvl1Tmp] -> rss_FaltInfoMng/84
  [bol_flgPwrTubPCBTempHiLvl2Tmp] -> rss_FaltInfoMng/85
  [bol_flgMotoTempHiLvl1Tmp] -> rss_FaltInfoMng/86
  [bol_flgMotoTempHiLvl2Tmp] -> rss_FaltInfoMng/87
  [bol_flgComFaltTmp] -> rss_FaltInfoMng/88
  [bol_flgMotoStallPermTmp] -> rss_FaltInfoMng/89
  [bol_flgMotoStallTmpTmp] -> rss_FaltInfoMng/90
  [bol_flgNoLdTmp] -> rss_FaltInfoMng/91
  [bol_flgBattPwrHiLvl1Tmp] -> rss_FaltInfoMng/92
  [bol_flgMotoSpdHiLvl1Tmp] -> rss_FaltInfoMng/93
  [bol_flgMotoSpdLoLvl1Tmp] -> rss_FaltInfoMng/94
  [bol_flgCtlBrdVltgLoLvl1Tmp] -> rss_FaltInfoMng/95
  [bol_flgCtlBrdVltgHiLvl1Tmp] -> rss_FaltInfoMng/96
  [bol_flgGDVltgLoLvl1Tmp] -> rss_FaltInfoMng/97
  [bol_flgGDVltgHiLvl1Tmp] -> rss_FaltInfoMng/98
  [bol_flgChipFaltTmp] -> rss_FaltInfoMng/99
  [bol_flgPhiSensFaltTmp] -> rss_FaltInfoMng/100
  [bol_flgPhCurrSensFaltTmp] -> rss_FaltInfoMng/101
  [bol_flgPwrTubPCBTempSensFaltTmp] -> rss_FaltInfoMng/102
  [bol_flgMotoTempSensFaltTmp] -> rss_FaltInfoMng/103
  [bol_flgBusOffFaltTmp] -> rss_FaltInfoMng/104
  [bol_flgCrashFaltTmp] -> rss_FaltInfoMng/105
  [bol_flgMosOpnCirFaltTmp] -> rss_FaltInfoMng/106
  rss_CtlBrdVltgLoLvl1Dia/3 -> [bol_flgCtlBrdVltgLoLvl1Tmp]
  rss_PhCurrHiLvl1Dia/3 -> [bol_flgPhCurrHiLvl1Tmp]
  rss_HWOvrCurrDia/3 -> [bol_flgHWOvrCurrTmp]
  rss_SplyVltgLoLvl1Dia/3 -> [bol_flgSplyVltgLoLvl1Tmp]
  rss_SplyVltgLoLvl2Dia/3 -> [bol_flgSplyVltgLoLvl2Tmp]
  rss_SplyVltgHiLvl1Dia/3 -> [bol_flgSplyVltgHiLvl1Tmp]
  rss_CtlBrdVltgHiLvl1Dia/3 -> [bol_flgCtlBrdVltgHiLvl1Tmp]
  rss_GDVltgLoLvl1Dia/3 -> [bol_flgGDVltgLoLvl1Tmp]
  rss_GDVltgHiLvl1Dia/3 -> [bol_flgGDVltgHiLvl1Tmp]
  rss_ChipFaltDia/3 -> [bol_flgChipFaltTmp]
  vrs_PhiSensFaltDia/4(bol_flgPhiSensFaltTmp) -> [bol_flgPhiSensFaltTmp]
  rss_PhCurrSensFaltDia/3 -> [bol_flgPhCurrSensFaltTmp]
  rss_BusOffFaltDia/3 -> [bol_flgBusOffFaltTmp]
  rss_CRASHFaltDia/3 -> [bol_flgCrashFaltTmp]
  rss_MosOpnCirFaltDia/3 -> [bol_flgMosOpnCirFaltTmp]
  rss_PwrTubPCBTempHiLvl1Dia/3 -> [bol_flgPwrTubPCBTempHiLvl1Tmp]
  rss_PwrTubPCBTempHiLvl2Dia/3 -> [bol_flgPwrTubPCBTempHiLvl2Tmp]
  rss_MotoTempHiLvl1Dia/3 -> [bol_flgMotoTempHiLvl1Tmp]
  rss_MotoTempHiLvl2Dia/3 -> [bol_flgMotoTempHiLvl2Tmp]
  rss_ComFaltDia/6 -> [bol_flgComFaltTmp]
  vrs_MotoStallDia/6(bol_flgMotoStallPermTmp) -> [bol_flgMotoStallPermTmp]
  vrs_MotoStallDia/7(bol_flgMotoStallTmpTmp) -> [bol_flgMotoStallTmpTmp]
  rss_NoLdDia/3 -> [bol_flgNoLdTmp]
  rss_BattPwrHiLvl1Dia/3 -> [bol_flgBattPwrHiLvl1Tmp]
  rss_MotoSpdHiLvl1Dia/3 -> [bol_flgMotoSpdHiLvl1Tmp]
  rss_MotoSpdLoLvl1Dia/3 -> [bol_flgMotoSpdLoLvl1Tmp]
  rss_PwrTubPCBTempSensFaltDia/3 -> [bol_flgPwrTubPCBTempSensFaltTmp]
  rss_MotoTempSensFaltDia/3 -> [bol_flgMotoTempSensFaltTmp]
  rss_FaltInfoMng/11 -> [busOBD_FaltStTmp]
  [busOBD_FaltStTmp] -> vrs_SlwTaskOut/9(busOBD_FaltStTmp)
  vrs_SlwTaskIn/49(bol_flgMosOpnCirFalt) -> [bol_flgMosOpnCirFalt]
  [u8_tPCBTempSubs] -> rss_PhCurrHiLvl1Dia/5

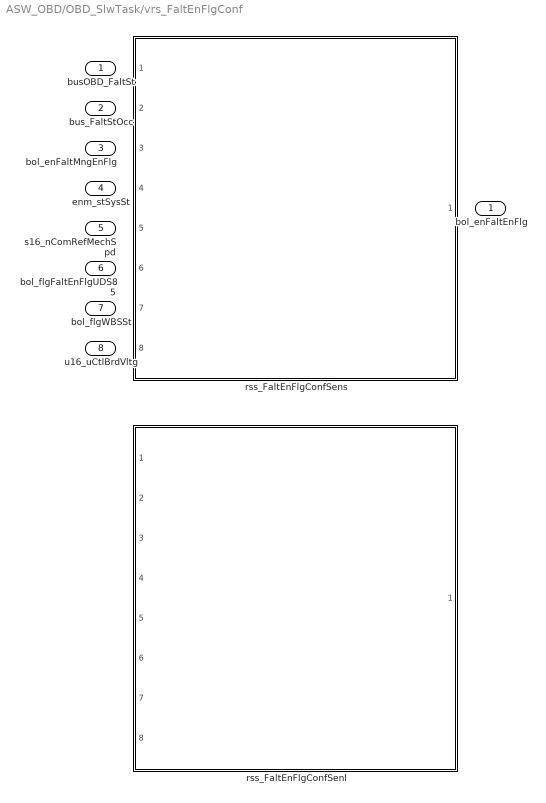
== system ASW_OBD/OBD_SlwTask/vrs_FaltEnFlgConf ==
  busOBD_FaltSt : Inport
  bus_FaltStOcc : Inport  Port=2
  bol_enFaltMngEnFlg : Inport  Port=3
  enm_stSysSt : Inport  Port=4
  s16_nComRefMechSpd : Inport  Port=5
  bol_flgFaltEnFlgUDS85 : Inport  Port=6
  bol_flgWBSSt : Inport  Port=7
  u16_uCtlBrdVltg : Inport  Port=8
  rss_FaltEnFlgConfSenl : Subsystem  VariantControl=cstSenlCtrlLbl  ReferencedSubsystem=rss_FaltEnFlgConfSenl
  rss_FaltEnFlgConfSens : Subsystem  VariantControl=cstSensCtrlLbl  ReferencedSubsystem=rss_FaltEnFlgConfSens
  bol_enFaltEnFlg : Outport

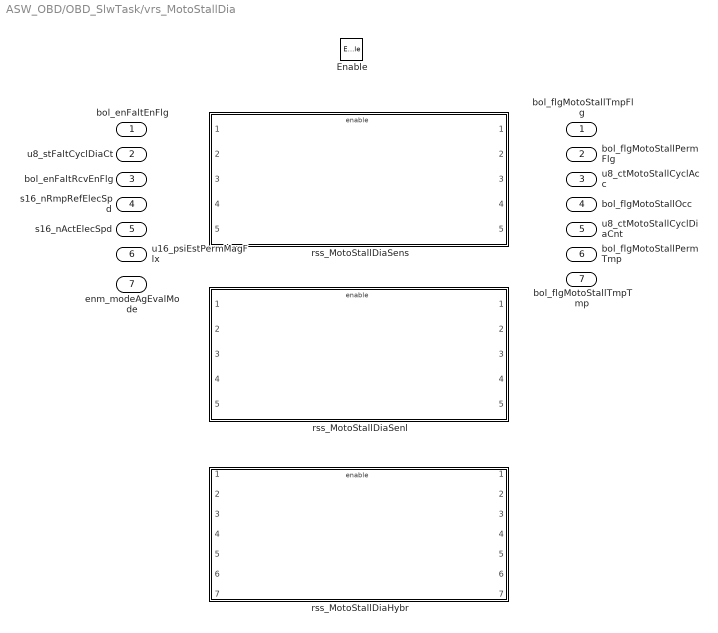
== system ASW_OBD/OBD_SlwTask/vrs_MotoStallDia ==
  bol_enFaltEnFlg : Inport
  u8_stFaltCyclDiaCt : Inport  Port=2
  bol_enFaltRcvEnFlg : Inport  Port=3
  s16_nRmpRefElecSpd : Inport  Port=4
  s16_nActElecSpd : Inport  Port=5
  u16_psiEstPermMagFlx : Inport  Port=6
  enm_modeAgEvalMode : Inport  Port=7
  Enable : EnablePort
  rss_MotoStallDiaHybr : Subsystem  VariantControl=cstHybrCtrlLbl  ReferencedSubsystem=rss_MotoStallDiaHybr
  rss_MotoStallDiaSenl : Subsystem  VariantControl=cstSenlCtrlLbl  ReferencedSubsystem=rss_MotoStallDiaSenl
  rss_MotoStallDiaSens : Subsystem  VariantControl=cstSensCtrlLbl  ReferencedSubsystem=rss_MotoStallDiaSens
  bol_flgMotoStallTmpFlg : Outport
  bol_flgMotoStallPermFlg : Outport  Port=2
  u8_ctMotoStallCyclAcc : Outport  Port=3
  bol_flgMotoStallOcc : Outport  Port=4
  u8_ctMotoStallCyclDiaCnt : Outport  Port=5
  bol_flgMotoStallPermTmp : Outport  Port=6
  bol_flgMotoStallTmpTmp : Outport  Port=7

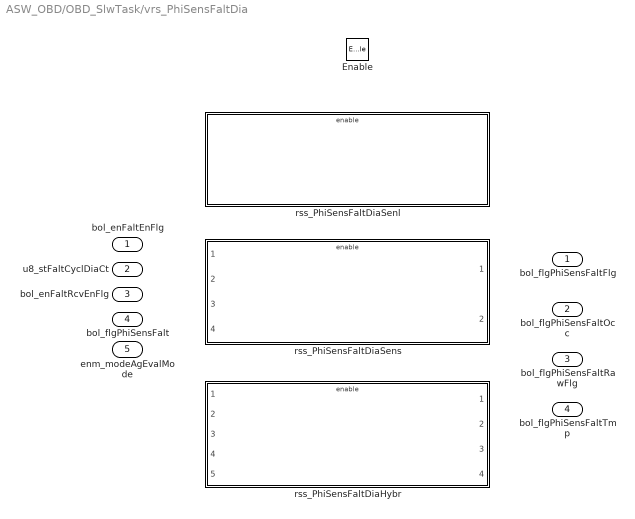
== system ASW_OBD/OBD_SlwTask/vrs_PhiSensFaltDia ==
  bol_enFaltEnFlg : Inport
  u8_stFaltCyclDiaCt : Inport  Port=2
  bol_enFaltRcvEnFlg : Inport  Port=3
  bol_flgPhiSensFalt : Inport  Port=4
  enm_modeAgEvalMode : Inport  Port=5
  Enable : EnablePort
  rss_PhiSensFaltDiaHybr : Subsystem  VariantControl=cstHybrCtrlLbl  ReferencedSubsystem=rss_PhiSensFaltDiaHybr
  rss_PhiSensFaltDiaSenl : Subsystem  VariantControl=cstSenlCtrlLbl
  rss_PhiSensFaltDiaSens : Subsystem  VariantControl=cstSensCtrlLbl  ReferencedSubsystem=rss_PhiSensFaltDiaSens
  bol_flgPhiSensFaltFlg : Outport
  bol_flgPhiSensFaltOcc : Outport  Port=2
  bol_flgPhiSensFaltRawFlg : Outport  Port=3
  bol_flgPhiSensFaltTmp : Outport  Port=4

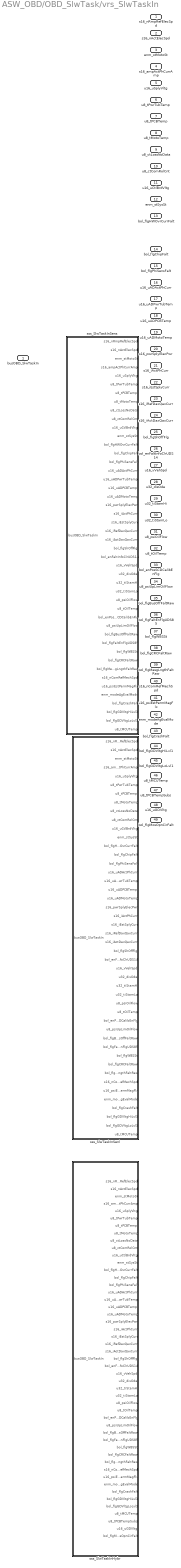
== system ASW_OBD/OBD_SlwTask/vrs_SlwTaskIn ==
  busOBD_SlwTaskIn : Inport
  sss_SlwTaskInHybr : Subsystem  VariantControl=cstHybrCtrlLbl
  sss_SlwTaskInSenl : Subsystem  VariantControl=cstSenlCtrlLbl
  sss_SlwTaskInSens : Subsystem  VariantControl=cstSensCtrlLbl
  s16_nRmpRefElecSpd : Outport
  s16_nActElecSpd : Outport  Port=2
  enm_stMotoSt : Outport  Port=3
  s16_ampActPhCurrAmp : Outport  Port=4
  u16_uSplyVltg : Outport  Port=5
  u8_tPwrTubTemp : Outport  Port=6
  u8_tPCBTemp : Outport  Port=7
  u8_tMotoTemp : Outport  Port=8
  u8_ctLossNoData : Outport  Port=9
  u8_ctComRolCnt : Outport  Port=10
  u16_uCtlBrdVltg : Outport  Port=11
  enm_stSysSt : Outport  Port=12
  bol_flgHWOvrCurrFalt : Outport  Port=13
  bol_flgChipFalt : Outport  Port=14
  bol_flgPhiSensFalt : Outport  Port=15
  u16_uADActPhCurr : Outport  Port=16
  u16_uADPwrTubTemp : Outport  Port=17
  u16_uADPCBTemp : Outport  Port=18
  u16_uADMotoTemp : Outport  Port=19
  s16_pwrSplyElecPwr : Outport  Port=20
  s16_iActPhCurr : Outport  Port=21
  s16_iEstSplyCurr : Outport  Port=22
  s16_iRefDaxQaxCurr : Outport  Port=23
  s16_iActDaxQaxCurr : Outport  Port=24
  bol_flgShOffFlg : Outport  Port=25
  bol_enFaltInfoClrUDS14 : Outport  Port=26
  u16_vVehSpd : Outport  Port=27
  u32_disOde : Outport  Port=28
  u32_tiStamHi : Outport  Port=29
  u32_tiStamLo : Outport  Port=30
  u8_psiOilFlow : Outport  Port=31
  u8_tOilTemp : Outport  Port=32
  bol_enPosSCDCalibEnFlg : Outport  Port=33
  u8_psiUpLimOilFlow : Outport  Port=34
  bol_flgBusOffFaltRaw : Outport  Port=35
  bol_flgFaltEnFlgUDS85 : Outport  Port=36
  bol_flgWBSSt : Outport  Port=37
  bol_flgCRCFaltRaw : Outport  Port=38
  bol_flgMesgLngthFaltRaw : Outport  Port=39
  s16_nComRefMechSpd : Outport  Port=40
  u16_psiEstPermMagFlx : Outport  Port=41
  enm_modeAgEvalMode : Outport  Port=42
  bol_flgCrashFalt : Outport  Port=43
  bol_flgGDVltgHiLvl1 : Outport  Port=44
  bol_flgGDVltgLoLvl1 : Outport  Port=45
  u8_tMCUTemp : Outport  Port=46
  u8_tPCBTempSubs : Outport  Port=47
  u16_uGDVltg : Outport  Port=48
  bol_flgMosOpnCirFalt : Outport  Port=49

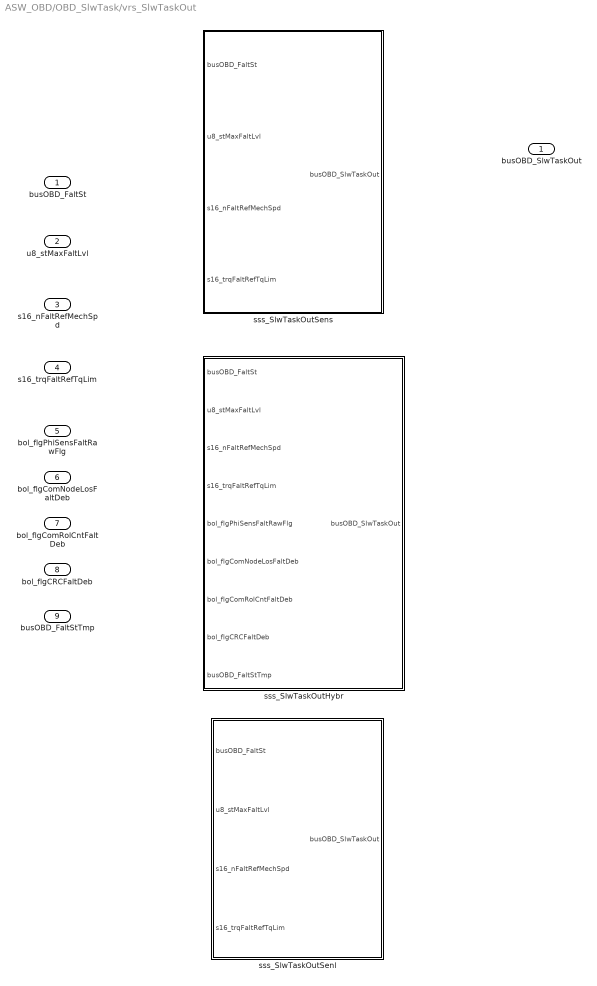
== system ASW_OBD/OBD_SlwTask/vrs_SlwTaskOut ==
  busOBD_FaltSt : Inport
  u8_stMaxFaltLvl : Inport  Port=2
  s16_nFaltRefMechSpd : Inport  Port=3
  s16_trqFaltRefTqLim : Inport  Port=4
  bol_flgPhiSensFaltRawFlg : Inport  Port=5
  bol_flgComNodeLosFaltDeb : Inport  Port=6
  bol_flgComRolCntFaltDeb : Inport  Port=7
  bol_flgCRCFaltDeb : Inport  Port=8
  busOBD_FaltStTmp : Inport  Port=9
  sss_SlwTaskOutHybr : Subsystem  VariantControl=cstHybrCtrlLbl
  sss_SlwTaskOutSenl : Subsystem  VariantControl=cstSenlCtrlLbl
  sss_SlwTaskOutSens : Subsystem  VariantControl=cstSensCtrlLbl
  busOBD_SlwTaskOut : Outport

== system ASW_OBD/OBD_SlwTask/vrs_PhiSensFaltDia/rss_PhiSensFaltDiaSenl ==
  Enable : EnablePort

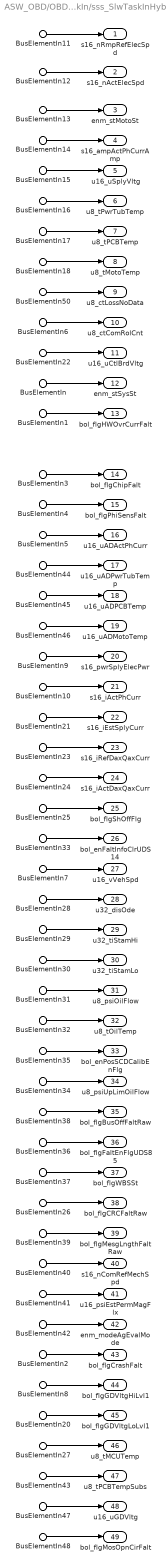
== system ASW_OBD/OBD_SlwTask/vrs_SlwTaskIn/sss_SlwTaskInHybr ==
  BusElementIn11 : Inport  PortName=busOBD_SlwTaskIn  Element=s16_nRmpRefElecSpd
  BusElementIn12 : Inport  PortName=busOBD_SlwTaskIn  Element=s16_nActElecSpd
  BusElementIn13 : Inport  PortName=busOBD_SlwTaskIn  Element=enm_stMotoSt
  BusElementIn14 : Inport  PortName=busOBD_SlwTaskIn  Element=s16_ampActPhCurrAmp
  BusElementIn15 : Inport  PortName=busOBD_SlwTaskIn  Element=u16_uSplyVltg
  BusElementIn16 : Inport  PortName=busOBD_SlwTaskIn  Element=u8_tPwrTubTemp
  BusElementIn17 : Inport  PortName=busOBD_SlwTaskIn  Element=u8_tPCBTemp
  BusElementIn18 : Inport  PortName=busOBD_SlwTaskIn  Element=u8_tMotoTemp
  BusElementIn22 : Inport  PortName=busOBD_SlwTaskIn  Element=u16_uCtlBrdVltg
  BusElementIn : Inport  PortName=busOBD_SlwTaskIn  Element=enm_stSysSt
  BusElementIn1 : Inport  PortName=busOBD_SlwTaskIn  Element=bol_flgHWOvrCurrFalt
  BusElementIn3 : Inport  PortName=busOBD_SlwTaskIn  Element=bol_flgChipFalt
  BusElementIn9 : Inport  PortName=busOBD_SlwTaskIn  Element=s16_pwrSplyElecPwr
  BusElementIn10 : Inport  PortName=busOBD_SlwTaskIn  Element=s16_iActPhCurr
  BusElementIn21 : Inport  PortName=busOBD_SlwTaskIn  Element=s16_iEstSplyCurr
  BusElementIn23 : Inport  PortName=busOBD_SlwTaskIn  Element=s16_iRefDaxQaxCurr
  BusElementIn24 : Inport  PortName=busOBD_SlwTaskIn  Element=s16_iActDaxQaxCurr
  BusElementIn25 : Inport  PortName=busOBD_SlwTaskIn  Element=bol_flgShOffFlg
  BusElementIn28 : Inport  PortName=busOBD_SlwTaskIn  Element=u32_disOde
  BusElementIn29 : Inport  PortName=busOBD_SlwTaskIn  Element=u32_tiStamHi
  BusElementIn30 : Inport  PortName=busOBD_SlwTaskIn  Element=u32_tiStamLo
  BusElementIn31 : Inport  PortName=busOBD_SlwTaskIn  Element=u8_psiOilFlow
  BusElementIn32 : Inport  PortName=busOBD_SlwTaskIn  Element=u8_tOilTemp
  BusElementIn34 : Inport  PortName=busOBD_SlwTaskIn  Element=u8_psiUpLimOilFlow
  BusElementIn35 : Inport  PortName=busOBD_SlwTaskIn  Element=bol_enPosSCDCalibEnFlg
  BusElementIn33 : Inport  PortName=busOBD_SlwTaskIn  Element=bol_enFaltInfoClrUDS14
  BusElementIn36 : Inport  PortName=busOBD_SlwTaskIn  Element=bol_flgFaltEnFlgUDS85
  BusElementIn37 : Inport  PortName=busOBD_SlwTaskIn  Element=bol_flgWBSSt
  BusElementIn38 : Inport  PortName=busOBD_SlwTaskIn  Element=bol_flgBusOffFaltRaw
  BusElementIn26 : Inport  PortName=busOBD_SlwTaskIn  Element=bol_flgCRCFaltRaw
  BusElementIn39 : Inport  PortName=busOBD_SlwTaskIn  Element=bol_flgMesgLngthFaltRaw
  BusElementIn40 : Inport  PortName=busOBD_SlwTaskIn  Element=s16_nComRefMechSpd
  BusElementIn41 : Inport  PortName=busOBD_SlwTaskIn  Element=u16_psiEstPermMagFlx
  BusElementIn4 : Inport  PortName=busOBD_SlwTaskIn  Element=bol_flgPhiSensFalt
  BusElementIn42 : Inport  PortName=busOBD_SlwTaskIn  Element=enm_modeAgEvalMode
  BusElementIn44 : Inport  PortName=busOBD_SlwTaskIn  Element=u16_uADPwrTubTemp
  BusElementIn45 : Inport  PortName=busOBD_SlwTaskIn  Element=u16_uADPCBTemp
  BusElementIn46 : Inport  PortName=busOBD_SlwTaskIn  Element=u16_uADMotoTemp
  BusElementIn5 : Inport  PortName=busOBD_SlwTaskIn  Element=u16_uADActPhCurr
  BusElementIn6 : Inport  PortName=busOBD_SlwTaskIn  Element=u8_ctComRolCnt
  BusElementIn7 : Inport  PortName=busOBD_SlwTaskIn  Element=u16_vVehSpd
  BusElementIn2 : Inport  PortName=busOBD_SlwTaskIn  Element=bol_flgCrashFalt
  BusElementIn8 : Inport  PortName=busOBD_SlwTaskIn  Element=bol_flgGDVltgHiLvl1
  BusElementIn20 : Inport  PortName=busOBD_SlwTaskIn  Element=bol_flgGDVltgLoLvl1
  BusElementIn27 : Inport  PortName=busOBD_SlwTaskIn  Element=u8_tMCUTemp
  BusElementIn43 : Inport  PortName=busOBD_SlwTaskIn  Element=u8_tPCBTempSubs
  BusElementIn47 : Inport  PortName=busOBD_SlwTaskIn  Element=u16_uGDVltg
  BusElementIn48 : Inport  PortName=busOBD_SlwTaskIn  Element=bol_flgMosOpnCirFalt
  BusElementIn50 : Inport  PortName=busOBD_SlwTaskIn  Element=u8_ctLossNoData
  s16_nRmpRefElecSpd : Outport
  s16_nActElecSpd : Outport  Port=2
  enm_stMotoSt : Outport  Port=3
  s16_ampActPhCurrAmp : Outport  Port=4
  u16_uSplyVltg : Outport  Port=5
  u8_tPwrTubTemp : Outport  Port=6
  u8_tPCBTemp : Outport  Port=7
  u8_tMotoTemp : Outport  Port=8
  u8_ctLossNoData : Outport  Port=9
  u8_ctComRolCnt : Outport  Port=10
  u16_uCtlBrdVltg : Outport  Port=11
  enm_stSysSt : Outport  Port=12
  bol_flgHWOvrCurrFalt : Outport  Port=13
  bol_flgChipFalt : Outport  Port=14
  bol_flgPhiSensFalt : Outport  Port=15
  u16_uADActPhCurr : Outport  Port=16
  u16_uADPwrTubTemp : Outport  Port=17
  u16_uADPCBTemp : Outport  Port=18
  u16_uADMotoTemp : Outport  Port=19
  s16_pwrSplyElecPwr : Outport  Port=20
  s16_iActPhCurr : Outport  Port=21
  s16_iEstSplyCurr : Outport  Port=22
  s16_iRefDaxQaxCurr : Outport  Port=23
  s16_iActDaxQaxCurr : Outport  Port=24
  bol_flgShOffFlg : Outport  Port=25
  bol_enFaltInfoClrUDS14 : Outport  Port=26
  u16_vVehSpd : Outport  Port=27
  u32_disOde : Outport  Port=28
  u32_tiStamHi : Outport  Port=29
  u32_tiStamLo : Outport  Port=30
  u8_psiOilFlow : Outport  Port=31
  u8_tOilTemp : Outport  Port=32
  bol_enPosSCDCalibEnFlg : Outport  Port=33
  u8_psiUpLimOilFlow : Outport  Port=34
  bol_flgBusOffFaltRaw : Outport  Port=35
  bol_flgFaltEnFlgUDS85 : Outport  Port=36
  bol_flgWBSSt : Outport  Port=37
  bol_flgCRCFaltRaw : Outport  Port=38
  bol_flgMesgLngthFaltRaw : Outport  Port=39
  s16_nComRefMechSpd : Outport  Port=40
  u16_psiEstPermMagFlx : Outport  Port=41
  enm_modeAgEvalMode : Outport  Port=42
  bol_flgCrashFalt : Outport  Port=43
  bol_flgGDVltgHiLvl1 : Outport  Port=44
  bol_flgGDVltgLoLvl1 : Outport  Port=45
  u8_tMCUTemp : Outport  Port=46
  u8_tPCBTempSubs : Outport  Port=47
  u16_uGDVltg : Outport  Port=48
  bol_flgMosOpnCirFalt : Outport  Port=49
  wires:
  BusElementIn41/1 -> u16_psiEstPermMagFlx/1
  BusElementIn40/1 -> s16_nComRefMechSpd/1
  BusElementIn39/1 -> bol_flgMesgLngthFaltRaw/1
  BusElementIn26/1 -> bol_flgCRCFaltRaw/1
  BusElementIn37/1 -> bol_flgWBSSt/1
  BusElementIn36/1 -> bol_flgFaltEnFlgUDS85/1
  BusElementIn38/1 -> bol_flgBusOffFaltRaw/1
  BusElementIn34/1 -> u8_psiUpLimOilFlow/1
  BusElementIn35/1 -> bol_enPosSCDCalibEnFlg/1
  BusElementIn32/1 -> u8_tOilTemp/1
  BusElementIn31/1 -> u8_psiOilFlow/1
  BusElementIn30/1 -> u32_tiStamLo/1
  BusElementIn29/1 -> u32_tiStamHi/1
  BusElementIn28/1 -> u32_disOde/1
  BusElementIn7/1 -> u16_vVehSpd/1
  BusElementIn33/1 -> bol_enFaltInfoClrUDS14/1
  BusElementIn25/1 -> bol_flgShOffFlg/1
  BusElementIn24/1 -> s16_iActDaxQaxCurr/1
  BusElementIn23/1 -> s16_iRefDaxQaxCurr/1
  BusElementIn21/1 -> s16_iEstSplyCurr/1
  BusElementIn10/1 -> s16_iActPhCurr/1
  BusElementIn9/1 -> s16_pwrSplyElecPwr/1
  BusElementIn46/1 -> u16_uADMotoTemp/1
  BusElementIn45/1 -> u16_uADPCBTemp/1
  BusElementIn44/1 -> u16_uADPwrTubTemp/1
  BusElementIn5/1 -> u16_uADActPhCurr/1
  BusElementIn3/1 -> bol_flgChipFalt/1
  BusElementIn1/1 -> bol_flgHWOvrCurrFalt/1
  BusElementIn/1 -> enm_stSysSt/1
  BusElementIn22/1 -> u16_uCtlBrdVltg/1
  BusElementIn18/1 -> u8_tMotoTemp/1
  BusElementIn6/1 -> u8_ctComRolCnt/1
  BusElementIn50/1 -> u8_ctLossNoData/1
  BusElementIn17/1 -> u8_tPCBTemp/1
  BusElementIn16/1 -> u8_tPwrTubTemp/1
  BusElementIn15/1 -> u16_uSplyVltg/1
  BusElementIn14/1 -> s16_ampActPhCurrAmp/1
  BusElementIn13/1 -> enm_stMotoSt/1
  BusElementIn12/1 -> s16_nActElecSpd/1
  BusElementIn11/1 -> s16_nRmpRefElecSpd/1
  BusElementIn4/1 -> bol_flgPhiSensFalt/1
  BusElementIn42/1 -> enm_modeAgEvalMode/1
  BusElementIn2/1 -> bol_flgCrashFalt/1
  BusElementIn8/1 -> bol_flgGDVltgHiLvl1/1
  BusElementIn20/1 -> bol_flgGDVltgLoLvl1/1
  BusElementIn27/1 -> u8_tMCUTemp/1
  BusElementIn43/1 -> u8_tPCBTempSubs/1
  BusElementIn47/1 -> u16_uGDVltg/1
  BusElementIn48/1 -> bol_flgMosOpnCirFalt/1

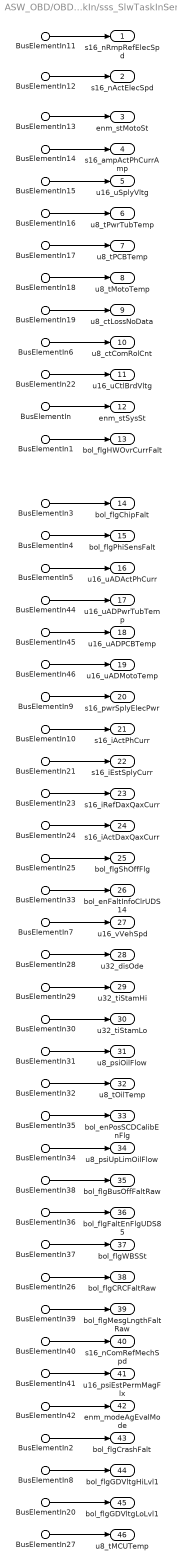
== system ASW_OBD/OBD_SlwTask/vrs_SlwTaskIn/sss_SlwTaskInSenl ==
  BusElementIn11 : Inport  PortName=busOBD_SlwTaskIn  Element=s16_nRmpRefElecSpd
  BusElementIn12 : Inport  PortName=busOBD_SlwTaskIn  Element=s16_nActElecSpd
  BusElementIn13 : Inport  PortName=busOBD_SlwTaskIn  Element=enm_stMotoSt
  BusElementIn14 : Inport  PortName=busOBD_SlwTaskIn  Element=s16_ampActPhCurrAmp
  BusElementIn15 : Inport  PortName=busOBD_SlwTaskIn  Element=u16_uSplyVltg
  BusElementIn16 : Inport  PortName=busOBD_SlwTaskIn  Element=u8_tPwrTubTemp
  BusElementIn17 : Inport  PortName=busOBD_SlwTaskIn  Element=u8_tPCBTemp
  BusElementIn18 : Inport  PortName=busOBD_SlwTaskIn  Element=u8_tMotoTemp
  BusElementIn22 : Inport  PortName=busOBD_SlwTaskIn  Element=u16_uCtlBrdVltg
  BusElementIn : Inport  PortName=busOBD_SlwTaskIn  Element=enm_stSysSt
  BusElementIn1 : Inport  PortName=busOBD_SlwTaskIn  Element=bol_flgHWOvrCurrFalt
  BusElementIn3 : Inport  PortName=busOBD_SlwTaskIn  Element=bol_flgChipFalt
  BusElementIn9 : Inport  PortName=busOBD_SlwTaskIn  Element=s16_pwrSplyElecPwr
  BusElementIn10 : Inport  PortName=busOBD_SlwTaskIn  Element=s16_iActPhCurr
  BusElementIn21 : Inport  PortName=busOBD_SlwTaskIn  Element=s16_iEstSplyCurr
  BusElementIn23 : Inport  PortName=busOBD_SlwTaskIn  Element=s16_iRefDaxQaxCurr
  BusElementIn24 : Inport  PortName=busOBD_SlwTaskIn  Element=s16_iActDaxQaxCurr
  BusElementIn25 : Inport  PortName=busOBD_SlwTaskIn  Element=bol_flgShOffFlg
  BusElementIn28 : Inport  PortName=busOBD_SlwTaskIn  Element=u32_disOde
  BusElementIn29 : Inport  PortName=busOBD_SlwTaskIn  Element=u32_tiStamHi
  BusElementIn30 : Inport  PortName=busOBD_SlwTaskIn  Element=u32_tiStamLo
  BusElementIn31 : Inport  PortName=busOBD_SlwTaskIn  Element=u8_psiOilFlow
  BusElementIn32 : Inport  PortName=busOBD_SlwTaskIn  Element=u8_tOilTemp
  BusElementIn34 : Inport  PortName=busOBD_SlwTaskIn  Element=u8_psiUpLimOilFlow
  BusElementIn35 : Inport  PortName=busOBD_SlwTaskIn  Element=bol_enPosSCDCalibEnFlg
  BusElementIn33 : Inport  PortName=busOBD_SlwTaskIn  Element=bol_enFaltInfoClrUDS14
  BusElementIn36 : Inport  PortName=busOBD_SlwTaskIn  Element=bol_flgFaltEnFlgUDS85
  BusElementIn37 : Inport  PortName=busOBD_SlwTaskIn  Element=bol_flgWBSSt
  BusElementIn38 : Inport  PortName=busOBD_SlwTaskIn  Element=bol_flgBusOffFaltRaw
  BusElementIn19 : Inport  PortName=busOBD_SlwTaskIn  Element=bol_flgComLosFaltRaw
  BusElementIn26 : Inport  PortName=busOBD_SlwTaskIn  Element=bol_flgCRCFaltRaw
  BusElementIn39 : Inport  PortName=busOBD_SlwTaskIn  Element=bol_flgMesgLngthFaltRaw
  BusElementIn40 : Inport  PortName=busOBD_SlwTaskIn  Element=s16_nComRefMechSpd
  BusElementIn41 : Inport  PortName=busOBD_SlwTaskIn  Element=u16_psiEstPermMagFlx
  BusElementIn4 : Inport  PortName=busOBD_SlwTaskIn  Element=bol_flgPhiSensFalt
  BusElementIn42 : Inport  PortName=busOBD_SlwTaskIn  Element=enm_modeAgEvalMode
  BusElementIn44 : Inport  PortName=busOBD_SlwTaskIn  Element=u16_uADPwrTubTemp
  BusElementIn45 : Inport  PortName=busOBD_SlwTaskIn  Element=u16_uADPCBTemp
  BusElementIn46 : Inport  PortName=busOBD_SlwTaskIn  Element=u16_uADMotoTemp
  BusElementIn5 : Inport  PortName=busOBD_SlwTaskIn  Element=u16_uADActPhCurr
  BusElementIn6 : Inport  PortName=busOBD_SlwTaskIn  Element=u8_ctComRolCnt
  BusElementIn7 : Inport  PortName=busOBD_SlwTaskIn  Element=u16_vVehSpd
  BusElementIn2 : Inport  PortName=busOBD_SlwTaskIn  Element=bol_flgCrashFalt
  BusElementIn8 : Inport  PortName=busOBD_SlwTaskIn  Element=bol_flgGDVltgHiLvl1
  BusElementIn20 : Inport  PortName=busOBD_SlwTaskIn  Element=bol_flgGDVltgLoLvl1
  BusElementIn27 : Inport  PortName=busOBD_SlwTaskIn  Element=u8_tMCUTemp
  s16_nRmpRefElecSpd : Outport
  s16_nActElecSpd : Outport  Port=2
  enm_stMotoSt : Outport  Port=3
  s16_ampActPhCurrAmp : Outport  Port=4
  u16_uSplyVltg : Outport  Port=5
  u8_tPwrTubTemp : Outport  Port=6
  u8_tPCBTemp : Outport  Port=7
  u8_tMotoTemp : Outport  Port=8
  u8_ctLossNoData : Outport  Port=9
  u8_ctComRolCnt : Outport  Port=10
  u16_uCtlBrdVltg : Outport  Port=11
  enm_stSysSt : Outport  Port=12
  bol_flgHWOvrCurrFalt : Outport  Port=13
  bol_flgChipFalt : Outport  Port=14
  bol_flgPhiSensFalt : Outport  Port=15
  u16_uADActPhCurr : Outport  Port=16
  u16_uADPwrTubTemp : Outport  Port=17
  u16_uADPCBTemp : Outport  Port=18
  u16_uADMotoTemp : Outport  Port=19
  s16_pwrSplyElecPwr : Outport  Port=20
  s16_iActPhCurr : Outport  Port=21
  s16_iEstSplyCurr : Outport  Port=22
  s16_iRefDaxQaxCurr : Outport  Port=23
  s16_iActDaxQaxCurr : Outport  Port=24
  bol_flgShOffFlg : Outport  Port=25
  bol_enFaltInfoClrUDS14 : Outport  Port=26
  u16_vVehSpd : Outport  Port=27
  u32_disOde : Outport  Port=28
  u32_tiStamHi : Outport  Port=29
  u32_tiStamLo : Outport  Port=30
  u8_psiOilFlow : Outport  Port=31
  u8_tOilTemp : Outport  Port=32
  bol_enPosSCDCalibEnFlg : Outport  Port=33
  u8_psiUpLimOilFlow : Outport  Port=34
  bol_flgBusOffFaltRaw : Outport  Port=35
  bol_flgFaltEnFlgUDS85 : Outport  Port=36
  bol_flgWBSSt : Outport  Port=37
  bol_flgCRCFaltRaw : Outport  Port=38
  bol_flgMesgLngthFaltRaw : Outport  Port=39
  s16_nComRefMechSpd : Outport  Port=40
  u16_psiEstPermMagFlx : Outport  Port=41
  enm_modeAgEvalMode : Outport  Port=42
  bol_flgCrashFalt : Outport  Port=43
  bol_flgGDVltgHiLvl1 : Outport  Port=44
  bol_flgGDVltgLoLvl1 : Outport  Port=45
  u8_tMCUTemp : Outport  Port=46
  wires:
  BusElementIn38/1 -> bol_flgBusOffFaltRaw/1
  BusElementIn34/1 -> u8_psiUpLimOilFlow/1
  BusElementIn35/1 -> bol_enPosSCDCalibEnFlg/1
  BusElementIn41/1 -> u16_psiEstPermMagFlx/1
  BusElementIn30/1 -> u32_tiStamLo/1
  BusElementIn26/1 -> bol_flgCRCFaltRaw/1
  BusElementIn7/1 -> u16_vVehSpd/1
  BusElementIn31/1 -> u8_psiOilFlow/1
  BusElementIn25/1 -> bol_flgShOffFlg/1
  BusElementIn10/1 -> s16_iActPhCurr/1
  BusElementIn27/1 -> u8_tMCUTemp/1
  BusElementIn20/1 -> bol_flgGDVltgLoLvl1/1
  BusElementIn19/1 -> u8_ctLossNoData/1
  BusElementIn39/1 -> bol_flgMesgLngthFaltRaw/1
  BusElementIn6/1 -> u8_ctComRolCnt/1
  BusElementIn40/1 -> s16_nComRefMechSpd/1
  BusElementIn23/1 -> s16_iRefDaxQaxCurr/1
  BusElementIn28/1 -> u32_disOde/1
  BusElementIn29/1 -> u32_tiStamHi/1
  BusElementIn17/1 -> u8_tPCBTemp/1
  BusElementIn12/1 -> s16_nActElecSpd/1
  BusElementIn33/1 -> bol_enFaltInfoClrUDS14/1
  BusElementIn2/1 -> bol_flgCrashFalt/1
  BusElementIn42/1 -> enm_modeAgEvalMode/1
  BusElementIn16/1 -> u8_tPwrTubTemp/1
  BusElementIn44/1 -> u16_uADPwrTubTemp/1
  BusElementIn22/1 -> u16_uCtlBrdVltg/1
  BusElementIn/1 -> enm_stSysSt/1
  BusElementIn5/1 -> u16_uADActPhCurr/1
  BusElementIn46/1 -> u16_uADMotoTemp/1
  BusElementIn45/1 -> u16_uADPCBTemp/1
  BusElementIn37/1 -> bol_flgWBSSt/1
  BusElementIn15/1 -> u16_uSplyVltg/1
  BusElementIn24/1 -> s16_iActDaxQaxCurr/1
  BusElementIn14/1 -> s16_ampActPhCurrAmp/1
  BusElementIn11/1 -> s16_nRmpRefElecSpd/1
  BusElementIn18/1 -> u8_tMotoTemp/1
  BusElementIn4/1 -> bol_flgPhiSensFalt/1
  BusElementIn13/1 -> enm_stMotoSt/1
  BusElementIn21/1 -> s16_iEstSplyCurr/1
  BusElementIn9/1 -> s16_pwrSplyElecPwr/1
  BusElementIn36/1 -> bol_flgFaltEnFlgUDS85/1
  BusElementIn3/1 -> bol_flgChipFalt/1
  BusElementIn32/1 -> u8_tOilTemp/1
  BusElementIn1/1 -> bol_flgHWOvrCurrFalt/1
  BusElementIn8/1 -> bol_flgGDVltgHiLvl1/1
